simulink model "sim_ecrd"  (R2013a)
settings: Solver=ode45  StartTime=0.0  StopTime=10  RelTol=1e-3
undefined symbols (not defined in the file or in its folder): sigbuilder_block
libraries: simulink x1
settings Model: Creator=Aleksandr  LastModifiedBy=Aleksandr

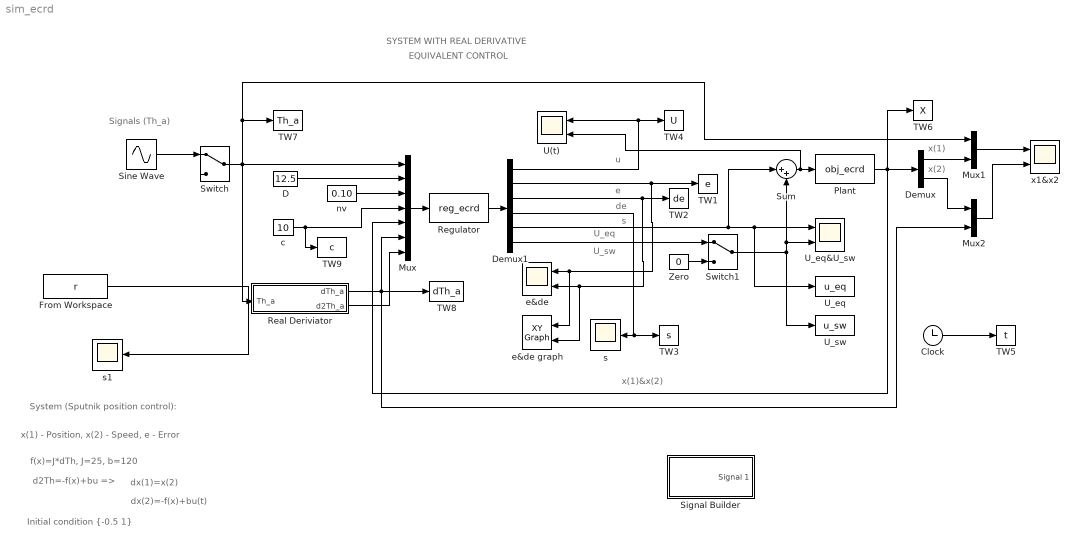
== system sim_ecrd ==
  note: U_sw
  note: U_eq
  note: EQUIVALENT CONTROL
  note: Initial condition {-0.5 1}
  note: f(x)=J*dTh, J=25, b=120
  note: dx(2)=-f(x)+bu(t)
  note: dx(1)=x(2)
  note: d2Th=-f(x)+bu =>
  note: System (Sputnik position control):
  note: x(1) - Position, x(2) - Speed,
      | e - Error
  note: s
  note: Signals (Th_a)
  note: x(1)&x(2)
  note: de
  note: e
  note: u
  note: x(2)
  note: x(1)
  note: SYSTEM WITH REAL DERIVATIVE
  " Switch" : ManualSwitch
  " Switch1" : ManualSwitch
  Clock : Clock
      settings: Decimation=15
  D : Constant  Value=12.5
  Demux : Demux  Outputs=2
  Demux1 : Demux  Outputs=6
  From Workspace : FromWorkspace  VariableName=r  SampleTime=0
  Mux : Mux  Inputs=7
  Mux1 : Mux  Inputs=2
  Mux2 : Mux  Inputs=2
  Plant : S-Function  FunctionName=obj_ecrd  EnableBusSupport=off
  Real Deriviator : Subsystem
  Regulator : S-Function  FunctionName=reg_ecrd  EnableBusSupport=off
  Signal Builder : Subsystem  Tag=STV Subsys  LoadFcn=sigbuilder_block('load',[437.25 117.75 550.5 394.5 ]);  StartFcn=sigbuilder_block('start');  StopFcn=sigbuilder_block('stop');  ClipboardFcn=sigbuilder_block('clipboard');  mask(Sigbuilder block){}
      mask help: Simulink:masks:SigbuilderBlock_MD
      mask init:
      | if ~strcmp(get_param(bdroot(gcbh),'SimulationStatus'),'stopped') tuvar = sigbuilder_block('maskInit'); end
      settings: CopyFcn=sigbuilder_block('copy');  DeleteFcn=sigbuilder_block('delete');  ModelCloseFcn=sigbuilder_block('modelClose');  PreSaveFcn=sigbuilder_block('preSave');  PauseFcn=sigbuilder_block('pause');  ContinueFcn=sigbuilder_block('continue');  NameChangeFcn=sigbuilder_block('namechange');  OpenFcn=sigbuilder_block('open',[437.6 199.2 550.4 400 ]);  CloseFcn=sigbuilder_block('close');
      mask Display: plot(0, 0, 100, 100,[2, 2, 32, 32, 2], [68, 8, 8, 68, 68],[32, 2], [38, 38], [32, 19, 2],[53, 60, 44], [32, 17, 17, 2],[16, 16, 31, 31]);txt = getActiveGroup(gcbh);text(2, 100, txt,'verticalAlignment', 'top');
  Sine Wave : Sin  SampleTime=0
  Sum : Sum  Inputs=|++
  TW1 : ToWorkspace  VariableName=e  SampleTime=-1
  TW2 : ToWorkspace  VariableName=de  SampleTime=-1
  TW3 : ToWorkspace  VariableName=s  SampleTime=-1
  TW4 : ToWorkspace  VariableName=U  SampleTime=-1
  TW5 : ToWorkspace  VariableName=t  SampleTime=-1
  TW6 : ToWorkspace  VariableName=X  SampleTime=-1
  TW7 : ToWorkspace  VariableName=Th_a  SampleTime=-1
  TW8 : ToWorkspace  VariableName=dTh_a  SampleTime=-1
  TW9 : ToWorkspace  VariableName=c  SampleTime=-1
  U(t) : Scope  NumInputPorts=2
      settings: YMin=-5~-5  YMax=5~5
  U_eq : ToWorkspace  VariableName=u_eq  SampleTime=-1
  U_eq&U_sw : Scope  NumInputPorts=2
      settings: TimeRange=3  YMin=-0.5~-1  YMax=1.5~4  SaveName=ScopeData4
  U_sw : ToWorkspace  VariableName=u_sw  SampleTime=-1
  "Zero " : Constant  Value=0
  c : Constant  Value=10
  e&de : Scope  NumInputPorts=2
      settings: TimeRange=20  YMin=-5~-5  YMax=5~5
  e&de graph : simulink/Sinks/XY Graph  xmin=-1  xmax=2  ymin=-0.75  ymax=1.5  st=.01
  nv : Constant  Value=0.10
  s : Scope
      settings: SaveName=ScopeData3
  s1 : Scope
      settings: SaveName=ScopeData5
  x1&x2 : Scope  NumInputPorts=2
      settings: TimeRange=3  YMin=-0.5~-1  YMax=1.5~4  SaveName=ScopeData2
  wires:
  " Switch"/1 -> Mux/1, TW7/1, Mux1/1, Real Deriviator/1(Th_a)
  Sine Wave/1 -> " Switch"/1
  D/1 -> Mux/2
  Mux/1 -> Regulator/1
  Regulator/1 -> Demux1/1
  Demux1/1 -> TW4/1, U(t)/1
  Demux1/2 -> TW1/1, e&de graph/1, e&de/1
  Demux1/3 -> TW2/1, e&de graph/2, e&de/2
  Demux1/4 -> TW3/1, s/1
  Plant/1 -> Mux/5, Demux/1, TW6/1
  Demux/1 -> Mux1/2
  Demux/2 -> Mux2/1
  Mux1/1 -> x1&x2/1
  Mux2/1 -> x1&x2/2
  Clock/1 -> TW5/1
  nv/1 -> Mux/3
  c/1 -> TW9/1, Mux/4
  Sum/1 -> U(t)/2, Plant/1
  Demux1/5 -> Sum/1, U_eq/1, U_eq&U_sw/1
  Demux1/6 -> " Switch1"/1
  " Switch1"/1 -> U_eq&U_sw/2, Sum/2, U_sw/1
  "Zero "/1 -> " Switch1"/2
  Real Deriviator/1(dTh_a) -> TW8/1, Mux2/2, Mux/6
  Real Deriviator/2(d2Th_a) -> Mux/7
  ? -> " Switch"/2
  From Workspace/1 -> s1/1

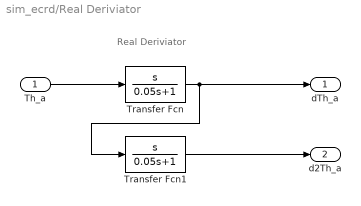
== system sim_ecrd/Real Deriviator ==
  note: Real Deriviator
  Th_a : Inport
  Transfer Fcn : TransferFcn  Numerator=[1 0]  Denominator=[0.05 1]
  Transfer Fcn1 : TransferFcn  Numerator=[1 0]  Denominator=[0.05 1]
  dTh_a : Outport
  d2Th_a : Outport  Port=2
  wires:
  Transfer Fcn/1 -> dTh_a/1, Transfer Fcn1/1
  Th_a/1 -> Transfer Fcn/1
  Transfer Fcn1/1 -> d2Th_a/1

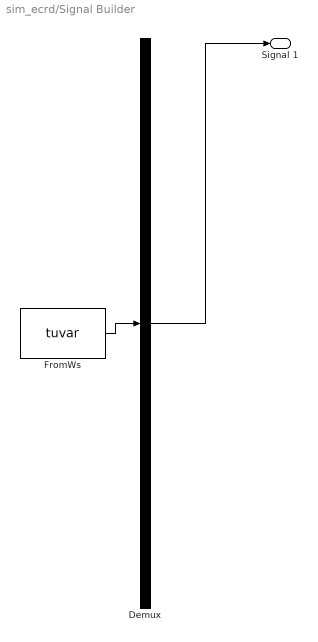
== system sim_ecrd/Signal Builder ==
  Demux : Demux  Tag=STV Demux  Outputs=1
  FromWs : FromWorkspace  Tag=STV FromWs  VariableName=tuvar  SampleTime=0
      SigBuilderData=|
      | common.afterFinalStr = 'Extrapolate'
      | common.sampleTime = 0
      | dataSet.timeRange = [0 10]
      | dataSet.name = 'Group 1'
      | sbobj.Groups.Name = 'Group 1'
      | sbobj.Groups.Signals.Name = 'Signal 1'
      | sbobj.Groups.Signals.XData = [0 4 4 6 6 10]
      | sbobj.Groups.Signals.YData = [0 0 1 1 0 0]
  Signal 1 : Outport  Tag=STV Outport
  wires:
  Demux/1 -> Signal 1/1
  FromWs/1 -> Demux/1
